simulink model "cambridge"  (R2023b)
settings: Solver=VariableStepAuto  StartTime=0.0  StopTime=15  FixedStep=0.0025  RelTol=1e-3
undefined symbols (not defined in the file or in its folder): body, ctrl, ground, planner, X, Y, Z
libraries: nesl_utility x71, sm_lib x43, slpidlib x24, simulink_extras x12, simulink x8, Contact_Forces_Lib x4, Parts_Lib x4, dspstat3 x1
(part 1 of 6)
settings Model: Creator=biorobotics  LastModifiedBy=Dayan-pc
settings SolverCC: AlgebraicLoopSolver=TrustRegion
settings DataIOCC: ReturnWorkspaceOutputs=off
settings OptimizationCC: ReuseModelBlockBuffer=off
settings DebuggingCC: UnconnectedInputMsg=warning  UnconnectedOutputMsg=warning  UnconnectedLineMsg=warning  ArithmeticOperatorsInVariantConditions=warning
settings ModelReferenceCC: EnableRefExpFcnMdlSchedulingChecks=on
settings SFSimCC: SimUseLocalCustomCode=off  CustomCodeUndefinedFunction=UseInterfaceOnly
settings RTWCC: RTWUseLocalCustomCode=off
settings DiagnosticsConfigSet: SimMechanicsRigidlyBoundBlock=none
settings ExplorerConfigSet: InternalSimMechanicsExplorerSettings="<ExplorerConfiguration><canonicalview>default</canonicalview><AnimationSetting><BasePlaybackSpeed>1.0</BasePlaybackSpeed><PlaybackSpeedFactor>1.0</PlaybackSpeedFactor></AnimationSetting><TilePanel><TileInfo><Tiles Columns=\"1\" Count=\"1\" Rows=\"1\"><Column Weight=\"1\"/><Row Weight=\"1\"/><Tile Height=\"1\" Width=\"1\" X=\"0\" Y=\"0\"/></Tiles></TileInfo><SceneInfo><SceneViewer><BGColor><R>0.60000002384185791</R><G>0.60000002384185791</G><B>0.60000002384185791</B></BGColor><Camera><DoPerspective>off</DoPerspective><Position><X>0</X><Y>-8.51131485710144098</Y><Z>0.265035197138786316</Z></Position><Center><X>0</X><Y>-1.14440917242664142e-07</Y><Z>0.265035197138786316</Z></Center><Up><X>0</X><Y>-0</Y><Z>1</Z></Up><ViewLimDist>1</ViewLimDist><YLim>8.00037523452157551</YLim><XLim>6.17999999999999972</XLim></Camera></SceneViewer></SceneInfo></TilePanel><MechEditorPanel><Cameras/><GfxPanelCameraMap/><VideoCreator><PlaybackSpeedRatio>1.0</PlaybackSpeedRatio><FrameRate>30</FrameRate><VideoFormat>Motion JPEG AVI</VideoFormat><FrameSize>auto</FrameSize></VideoCreator></MechEditorPanel></ExplorerConfiguration>"

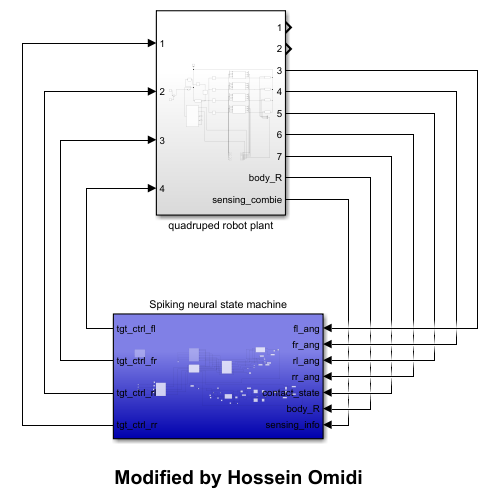
[thumbnail: Simulink's stored preview of the top-level diagram]
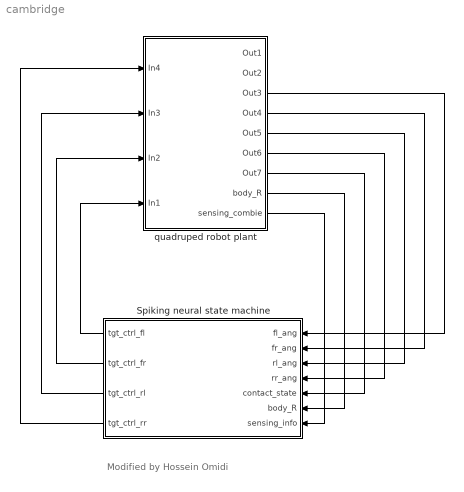
== system cambridge ==
  note: Modified by Hossein Omidi
  Spiking neural state machine : Subsystem
  quadruped robot plant : Subsystem
  wires:
  Spiking neural state machine/1(tgt_ctrl_fl) -> quadruped robot plant/4(In1)
  Spiking neural state machine/2(tgt_ctrl_fr) -> quadruped robot plant/3(In2)
  Spiking neural state machine/3(tgt_ctrl_rl) -> quadruped robot plant/2(In3)
  Spiking neural state machine/4(tgt_ctrl_rr) -> quadruped robot plant/1(In4)
  quadruped robot plant/3(Out3) -> Spiking neural state machine/1(fl_ang)
  quadruped robot plant/4(Out4) -> Spiking neural state machine/2(fr_ang)
  quadruped robot plant/5(Out5) -> Spiking neural state machine/3(rl_ang)
  quadruped robot plant/6(Out6) -> Spiking neural state machine/4(rr_ang)
  quadruped robot plant/7(Out7) -> Spiking neural state machine/5(contact_state)
  quadruped robot plant/8(body_R) -> Spiking neural state machine/6(body_R)
  quadruped robot plant/9(sensing_combie) -> Spiking neural state machine/7(sensing_info)

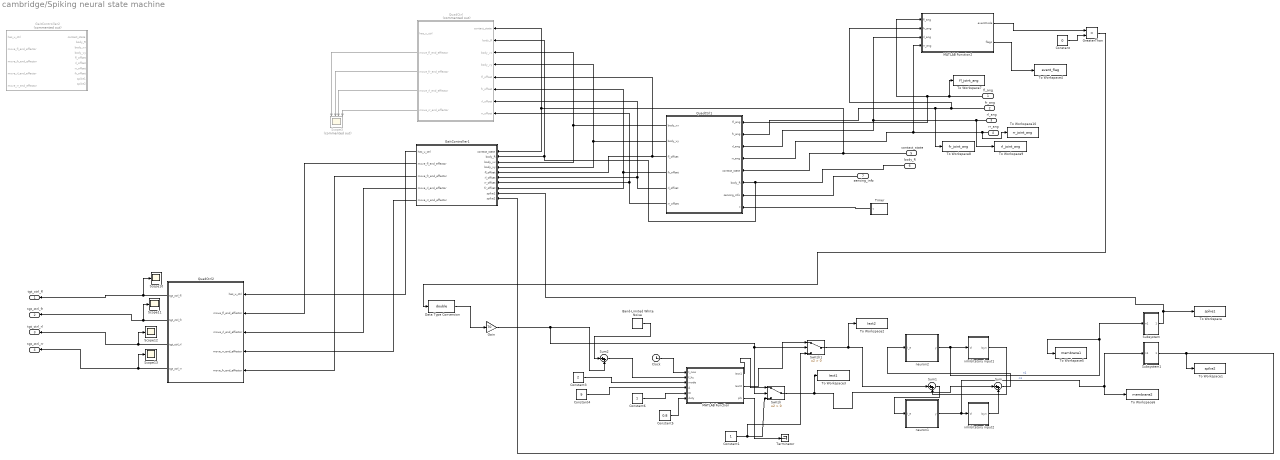
== system cambridge/Spiking neural state machine ==
  fl_ang : Inport
  fr_ang : Inport  Port=2
  rl_ang : Inport  Port=3
  rr_ang : Inport  Port=4
  contact_state : Inport  Port=5
  body_R : Inport  Port=6
  sensing_info : Inport  Port=7
  Band-Limited White Noise : simulink/Sources/Band-Limited White Noise  Cov=[0.1]  Ts=0.1  seed=[23341]
  Clock : Clock
  Constant : Constant  Value=0
  Constant1 : Constant
  Constant3 : Constant  Value=2
  Constant4 : Constant  Value=9
  Constant5 : Constant  Value=0.8
  Constant6 : Constant
  Data Type Conversion : DataTypeConversion  OutDataTypeStr=double  SaturateOnIntegerOverflow=off  RndMeth=Floor
  Gain : Gain  Gain=70
  GaitController1 : Stateflow chart  InitFcn=|  TreatAsAtomicUnit=on
      | % tick timers
      | timer  = uint16(0);
      | timer2 = uint16(0);
      | 
      | % shoulder offsets (body frame)
      | fl_offset = [ body.shoulder_distance;  body.y_length/2 + body.shoulder_size/2; 0 ];
      | fr_offset = [ body.shoulder_distance; -body.y_length/2 - body.shoulder_size/2; 0 ];
      | rl_offset = [-body.shoulder_distance;  body.y_length/2 + body.shoulder_size/2; 0 ];
      | rr_offset = [-body.shoulder_distance; -body.y_length/2 - body.shoulder_size/2; 0 ];
      | 
      | % nominal virtual legs (body frame)
      | vleg1_n = [0;0;planner.stand_height];
      | vleg2_n = [0;0;planner.stand_height];
      | 
      | % swing timing in ticks
      | t_leg    = uint16(planner.leg_swing_time);
      | half_leg = uint16(floor(double(t_leg)/2));
      | 
      | % safe IK inputs on first tick
      | mv_fl = vleg1_n; mv_rr = vleg1_n;
      | mv_fr = vleg2_n; mv_rl = vleg2_n;
      | has_u_ctrl = [1;1;1;1];
  GaitController2 : Stateflow chart  Commented=on  InitFcn=|  TreatAsAtomicUnit=on
      | % tick timers
      | timer  = uint16(0);
      | timer2 = uint16(0);
      | 
      | % shoulder offsets (body frame)
      | fl_offset = [ body.shoulder_distance;  body.y_length/2 + body.shoulder_size/2; 0 ];
      | fr_offset = [ body.shoulder_distance; -body.y_length/2 - body.shoulder_size/2; 0 ];
      | rl_offset = [-body.shoulder_distance;  body.y_length/2 + body.shoulder_size/2; 0 ];
      | rr_offset = [-body.shoulder_distance; -body.y_length/2 - body.shoulder_size/2; 0 ];
      | 
      | % nominal virtual legs (body frame)
      | vleg1_n = [0;0;planner.stand_height];
      | vleg2_n = [0;0;planner.stand_height];
      | 
      | % swing timing in ticks
      | t_leg    = uint16(planner.leg_swing_time);
      | half_leg = uint16(floor(double(t_leg)/2));
      | 
      | % safe IK inputs on first tick
      | mv_fl = vleg1_n; mv_rr = vleg1_n;
      | mv_fr = vleg2_n; mv_rl = vleg2_n;
      | has_u_ctrl = [1;1;1;1];
  GreaterThan : RelationalOperator  Operator=>  OutDataTypeStr=boolean  RndMeth=Simplest  InputSameDT=off
  MATLAB Function : MATLAB Function  TreatAsAtomicUnit=on
  MATLAB Function2 : MATLAB Function  TreatAsAtomicUnit=on
  QuadCtrl : MATLAB Function  Commented=on  TreatAsAtomicUnit=on  SystemSampleTime=0.0025
  QuadCtrl1 : MATLAB Function  TreatAsAtomicUnit=on  SystemSampleTime=0.0025
  QuadCtrl2 : MATLAB Function  TreatAsAtomicUnit=on  SystemSampleTime=0.0025
  Scope{10..13} (4 alike) : Scope
  Scope3 : Scope  Commented=on  NumInputPorts=4
  Subsystem : Subsystem
  Subsystem1 : Subsystem
  Sum : Sum  Inputs=|++
  Sum1 : Sum  Inputs=|++
  Sum2 : Sum  Inputs=|++
  Switch : Switch  Criteria=u2 > Threshold  SaturateOnIntegerOverflow=off  InputSameDT=off
  Switch1 : Switch  Criteria=u2 > Threshold  SaturateOnIntegerOverflow=off  InputSameDT=off
  Terminator : Terminator
  Timer : Subsystem
  To Workspace : ToWorkspace  VariableName=spike1  SaveFormat=Timeseries  SampleTime=-1
  To Workspace1 : ToWorkspace  VariableName=spike2  SaveFormat=Timeseries  SampleTime=-1
  To Workspace10 : ToWorkspace  VariableName=rr_joint_ang  SaveFormat=Timeseries  SampleTime=-1
  To Workspace2 : ToWorkspace  VariableName=Iext2  SaveFormat=Timeseries  SampleTime=-1
  To Workspace3 : ToWorkspace  VariableName=Iext1  SaveFormat=Timeseries  SampleTime=-1
  To Workspace4 : ToWorkspace  VariableName=event_flag  SaveFormat=Timeseries  SampleTime=-1
  To Workspace5 : ToWorkspace  VariableName=membrane1  SaveFormat=Timeseries  SampleTime=-1
  To Workspace6 : ToWorkspace  VariableName=membrane2  SaveFormat=Timeseries  SampleTime=-1
  To Workspace7 : ToWorkspace  VariableName=fl_joint_ang  SaveFormat=Timeseries  SampleTime=-1
  To Workspace8 : ToWorkspace  VariableName=fr_joint_ang  SaveFormat=Timeseries  SampleTime=-1
  To Workspace9 : ToWorkspace  VariableName=rl_joint_ang  SaveFormat=Timeseries  SampleTime=-1
  inhibitatory input1 : Subsystem
  inhibitatory input2 : Subsystem
  neuron1 : Subsystem
  neuron2 : Subsystem
  tgt_ctrl_fl : Outport  VectorParamsAs1DForOutWhenUnconnected=off
  tgt_ctrl_fr : Outport  Port=2  VectorParamsAs1DForOutWhenUnconnected=off
  tgt_ctrl_rl : Outport  Port=3  VectorParamsAs1DForOutWhenUnconnected=off
  tgt_ctrl_rr : Outport  Port=4  VectorParamsAs1DForOutWhenUnconnected=off
  wires:
  Timer/1(t) -> QuadCtrl1/8(t)
  fl_ang/1 -> To Workspace7/1, MATLAB Function2/1(fl_ang), QuadCtrl1/1(fl_ang)
  fr_ang/1 -> To Workspace8/1, QuadCtrl1/2(fr_ang), MATLAB Function2/2(fr_ang)
  rl_ang/1 -> To Workspace9/1, MATLAB Function2/3(rl_ang), QuadCtrl1/3(rl_ang)
  rr_ang/1 -> To Workspace10/1, MATLAB Function2/4(rr_ang), QuadCtrl1/4(rr_ang)
  sensing_info/1 -> QuadCtrl1/7(sensing_info)
  QuadCtrl2/1(tgt_ctrl_fl) -> Scope10/1, tgt_ctrl_fl/1
  QuadCtrl2/2(tgt_ctrl_fr) -> Scope11/1, tgt_ctrl_fr/1
  QuadCtrl2/3(tgt_ctrl_rl) -> Scope12/1, tgt_ctrl_rl/1
  QuadCtrl2/4(tgt_ctrl_rr) -> Scope13/1, tgt_ctrl_rr/1
  contact_state/1 -> QuadCtrl/1(contact_state), GaitController1/1(contact_state), QuadCtrl1/5(contact_state)
  body_R/1 -> QuadCtrl/2(body_R), GaitController1/2(body_R), QuadCtrl1/6(body_R)
  QuadCtrl1/1(body_vx) -> QuadCtrl/3(body_vx), GaitController1/3(body_vx)
  QuadCtrl1/2(body_vy) -> QuadCtrl/4(body_vy), GaitController1/4(body_vy)
  QuadCtrl1/3(fl_offset) -> QuadCtrl/5(fl_offset), GaitController1/5(fl_offset)
  QuadCtrl1/5(rl_offset) -> QuadCtrl/7(rl_offset), GaitController1/6(rl_offset)
  QuadCtrl1/6(rr_offset) -> QuadCtrl/8(rr_offset), GaitController1/7(rr_offset)
  QuadCtrl1/4(fr_offset) -> QuadCtrl/6(fr_offset), GaitController1/8(fr_offset)
  GaitController1/1(has_u_ctrl) -> QuadCtrl2/1(has_u_ctrl)
  GaitController1/2(move_fl_end_effector) -> QuadCtrl2/2(move_fl_end_effector)
  GaitController1/3(move_fr_end_effector) -> QuadCtrl2/5(move_fr_end_effector)
  GaitController1/4(move_rl_end_effector) -> QuadCtrl2/3(move_rl_end_effector)
  GaitController1/5(move_rr_end_effector) -> QuadCtrl2/4(move_rr_end_effector)
  QuadCtrl/2(move_fl_end_effector) -> Scope3/1
  QuadCtrl/3(move_fr_end_effector) -> Scope3/2
  QuadCtrl/4(move_rl_end_effector) -> Scope3/3
  QuadCtrl/5(move_rr_end_effector) -> Scope3/4
  MATLAB Function2/2(flags) -> To Workspace4/1
  Constant3/1 -> MATLAB Function/3(mode)
  Gain/1 -> Sum2/2, Switch1/2, Switch/2
  Clock/1 -> MATLAB Function/1(t_now)
  inhibitatory input2/1(Isyn) -> Sum/2
  Constant5/1 -> MATLAB Function/6(duty)
  inhibitatory input1/1(Isyn) -> Sum1/2
  Constant4/1 -> MATLAB Function/4(A)
  Constant6/1 -> MATLAB Function/5(I0)
  Subsystem1/1(spike2) -> To Workspace1/1, GaitController1/10(spike2)
  Sum/1 -> neuron2/1(I_e)
  neuron2/1(y) -> Subsystem/1(n1), To Workspace5/1, inhibitatory input1/1(Vi)  "n1"
  MATLAB Function/2(Iext2) -> Switch1/1
  neuron1/1(y) -> Subsystem1/1(n1), To Workspace6/1, inhibitatory input2/1(Vi)  "n1"
  Sum1/1 -> neuron1/1(I_e)
  MATLAB Function/1(Iext1) -> Switch/1
  MATLAB Function2/1(eventCode) -> GreaterThan/1
  Constant/1 -> GreaterThan/2
  Data Type Conversion/1 -> Gain/1
  GreaterThan/1 -> Data Type Conversion/1
  Switch/1 -> To Workspace3/1, Sum/1
  Constant1/1 -> Switch1/3, Switch/3
  Switch1/1 -> To Workspace2/1, Sum1/1
  Subsystem/1(Out1) -> To Workspace/1, GaitController1/9(spike1)
  Band-Limited White Noise/1 -> Sum2/1
  Sum2/1 -> MATLAB Function/2(f_hz)
  MATLAB Function/3(phi) -> Terminator/1

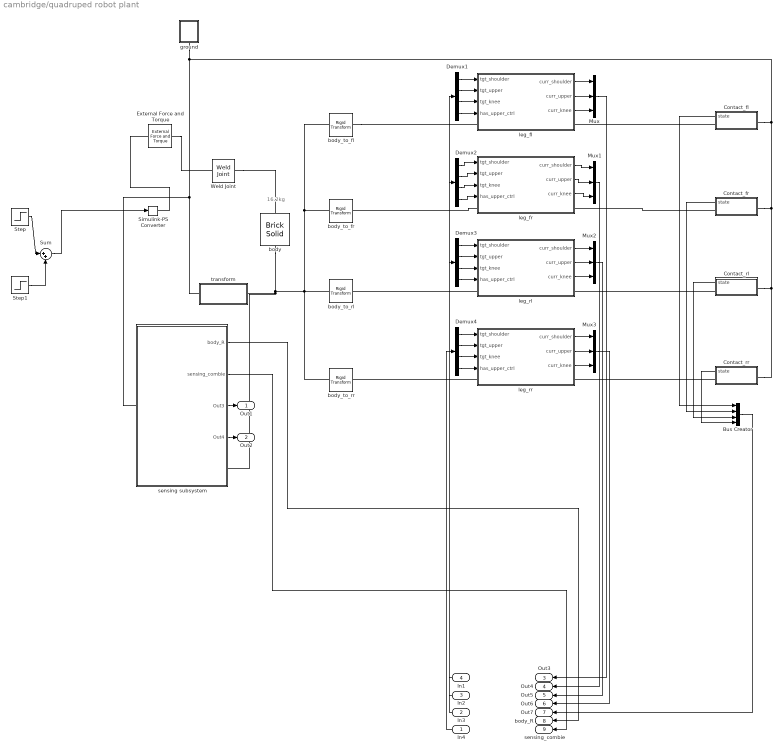
== system cambridge/quadruped robot plant ==
  note: 16.2kg
  In4 : Inport
  In3 : Inport  Port=2
  In2 : Inport  Port=3
  In1 : Inport  Port=4
  Bus Creator : BusCreator  Inputs=4
  Contact_fl : Subsystem
  Contact_fr : Subsystem
  Contact_rl : Subsystem
  Contact_rr : Subsystem
  Demux{1..4} (4 alike) : Demux
  External Force and Torque : sm_lib/Forces and Torques/External Force and Torque  ForceResolutionFrame=AttachedFrame  EnableForceX=on  EnableForceY=off  EnableForceZ=off  EnableForce=off  TorqueResolutionFrame=AttachedFrame  EnableTorqueX=off  EnableTorqueY=off  EnableTorqueZ=off  EnableTorque=off
  Mux{,1..3} (4 alike) : Mux  Inputs=3
  Simulink-PS Converter : nesl_utility/Simulink-PS Converter  PhysicalDomain=network_engine_domain  SubClassName=ps_input  LeftPortType=input  RightPortType=output  PseudoPeriodic=off  Frequencies=[]  NoiseDistribution=none  NoiseParameters=[]  Unit=1  AffineConversion=off  FilteringAndDerivatives=provide  SimscapeFilterOrder=1  InputFilterTimeConstant=0.001  UdotUserProvided=0
  Step : Step  Time=5  After=100  SampleTime=0
  Step1 : Step  Time=5.1  After=-100  SampleTime=0
  Sum : Sum  Inputs=|++
  Weld Joint : sm_lib/Joints/Weld Joint  JointMode=Normal  SenseConstraintForce=off  SenseConstraintForceX=off  SenseConstraintForceY=off  SenseConstraintForceZ=off  SenseConstraintTorque=off  SenseConstraintTorqueX=off  SenseConstraintTorqueY=off  SenseConstraintTorqueZ=off  SenseTotalForce=off  SenseTotalForceX=off  SenseTotalForceY=off  SenseTotalForceZ=off  SenseTotalTorque=off  SenseTotalTorqueX=off  SenseTotalTorqueY=off  SenseTotalTorqueZ=off  CompositeWrenchDir=FollowerOnBase  CompositeWrenchFrame=BaseFrame
  body : sm_lib/Body Elements/Brick Solid  GraphicAmbientColor=[0.15 0.15 0.15 1.0]  BasedOnType=Density  BrickDimensions=[body.x_length body.y_length body.z_length]  BrickDimensionsUnits=m  CenterOfMass=[0 0 0]  CenterOfMassUnits=m  GraphicDiffuseColor=[1.0 0.0 0.2]  Density=600  DensityUnits=kg/(m^3)  DoExposeReferenceFrame=on  GraphicEmissiveColor=[0.0 0.0 0.0 1.0]  ExportEntireGeometry=off  SerializedFrames=<Frames><Frame><Id>Frame2</Id><Value><Name>force</Name><Origin><Source>CenterOfMassFrame</Source><FeatureName></FeatureName></Origin><PrimaryAxis><DefinedDirection>+Z</DefinedDirection><Source>ReferenceFrame</Source><SourceDirection>+Z</SourceDirection><FeatureName></FeatureName></PrimaryAxis><SecondaryAxis><DefinedDirection>+X</DefinedDirection><Source>ReferenceFrame</Source><SourceDirection>+X</SourceDirection><FeatureName></FeatureName></SecondaryAxis></Value></Frame></Frames>  MarkerShape=Sphere  MarkerSize=10  GraphicType=FromGeometry  InertiaType=CalculateFromGeometry  Mass=8.6  MassUnits=kg  MomentsOfInertia=[1 1 1]  MomentsOfInertiaUnits=kg*m^2  GraphicOpacity=1.0  ProductsOfInertia=[0 0 0]  ProductsOfInertiaUnits=kg*m^2  GraphicShininess=75  GraphicSpecularColor=[0.5 0.5 0.5 1.0]  GraphicVisPropType=SimpleVisualProperties
  body_to_fl : sm_lib/Frames and Transforms/Rigid Transform  TranslationMethod=Cartesian  TranslationStandardOffset=0  TranslationStandardOffsetUnits=m  TranslationStandardAxis=+Z  TranslationCartesianOffset=[body.shoulder_distance body.y_length/2+body.shoulder_size/2 0]  TranslationCartesianOffsetUnits=m  TranslationROffset=0  TranslationROffsetUnits=m  TranslationZOffset=0  TranslationZOffsetUnits=m  TranslationThetaOffset=0  TranslationThetaOffsetUnits=deg  RotationMethod=AlignedAxes  RotationAngleUnits=deg  RotationStandardAxis=+Z  RotationAngle=0.0  RotationArbitraryAxis=[0 0 1]  FollAlignAxisA=+Z  BaseAlignAxisA=+X  FollAlignAxisB=+X  BaseAlignAxisB=-Z  RotationSequenceAxes=FollowerAxes  RotationSequence=XYX  RotationSequenceAngles=[0 0 0]  RotationSequenceAnglesUnits=deg  RotationMatrix=[1 0 0; 0 1 0; 0 0 1]  Quaternion=[1 0 0 0]
  body_to_fr : sm_lib/Frames and Transforms/Rigid Transform  TranslationMethod=Cartesian  TranslationStandardOffset=0  TranslationStandardOffsetUnits=m  TranslationStandardAxis=+Z  TranslationCartesianOffset=[body.shoulder_distance -body.y_length/2-body.shoulder_size/2 0]  TranslationCartesianOffsetUnits=m  TranslationROffset=0  TranslationROffsetUnits=m  TranslationZOffset=0  TranslationZOffsetUnits=m  TranslationThetaOffset=0  TranslationThetaOffsetUnits=deg  RotationMethod=AlignedAxes  RotationAngleUnits=deg  RotationStandardAxis=+Z  RotationAngle=0.0  RotationArbitraryAxis=[0 0 1]  FollAlignAxisA=+Z  BaseAlignAxisA=+X  FollAlignAxisB=+X  BaseAlignAxisB=-Z  RotationSequenceAxes=FollowerAxes  RotationSequence=XYX  RotationSequenceAngles=[0 0 0]  RotationSequenceAnglesUnits=deg  RotationMatrix=[1 0 0; 0 1 0; 0 0 1]  Quaternion=[1 0 0 0]
  body_to_rl : sm_lib/Frames and Transforms/Rigid Transform  TranslationMethod=Cartesian  TranslationStandardOffset=0  TranslationStandardOffsetUnits=m  TranslationStandardAxis=+Z  TranslationCartesianOffset=[-body.shoulder_distance body.y_length/2+body.shoulder_size/2 0]  TranslationCartesianOffsetUnits=m  TranslationROffset=0  TranslationROffsetUnits=m  TranslationZOffset=0  TranslationZOffsetUnits=m  TranslationThetaOffset=0  TranslationThetaOffsetUnits=deg  RotationMethod=AlignedAxes  RotationAngleUnits=deg  RotationStandardAxis=+Z  RotationAngle=0.0  RotationArbitraryAxis=[0 0 1]  FollAlignAxisA=+Z  BaseAlignAxisA=+X  FollAlignAxisB=+X  BaseAlignAxisB=-Z  RotationSequenceAxes=FollowerAxes  RotationSequence=XYX  RotationSequenceAngles=[0 0 0]  RotationSequenceAnglesUnits=deg  RotationMatrix=[1 0 0; 0 1 0; 0 0 1]  Quaternion=[1 0 0 0]
  body_to_rr : sm_lib/Frames and Transforms/Rigid Transform  TranslationMethod=Cartesian  TranslationStandardOffset=0  TranslationStandardOffsetUnits=m  TranslationStandardAxis=+Z  TranslationCartesianOffset=[-body.shoulder_distance -body.y_length/2-body.shoulder_size/2 0]  TranslationCartesianOffsetUnits=m  TranslationROffset=0  TranslationROffsetUnits=m  TranslationZOffset=0  TranslationZOffsetUnits=m  TranslationThetaOffset=0  TranslationThetaOffsetUnits=deg  RotationMethod=AlignedAxes  RotationAngleUnits=deg  RotationStandardAxis=+Z  RotationAngle=0.0  RotationArbitraryAxis=[0 0 1]  FollAlignAxisA=+Z  BaseAlignAxisA=+X  FollAlignAxisB=+X  BaseAlignAxisB=-Z  RotationSequenceAxes=FollowerAxes  RotationSequence=XYX  RotationSequenceAngles=[0 0 0]  RotationSequenceAnglesUnits=deg  RotationMatrix=[1 0 0; 0 1 0; 0 0 1]  Quaternion=[1 0 0 0]
  ground : Subsystem
  leg_fl : Subsystem
  leg_fr : Subsystem
  leg_rl : Subsystem
  leg_rr : Subsystem
  "sensing subsystem " : Subsystem
  transform : Subsystem
  Out1 : Outport
  Out2 : Outport  Port=2
  Out3 : Outport  Port=3
  Out4 : Outport  Port=4
  Out5 : Outport  Port=5
  Out6 : Outport  Port=6
  Out7 : Outport  Port=7
  body_R : Outport  Port=8
  sensing_combie : Outport  Port=9
  wires:
  Bus Creator/1 -> Out7/1
  Demux2/1 -> leg_fr/1(tgt_shoulder)
  Demux1/2 -> leg_fl/2(tgt_upper)
  Demux2/3 -> leg_fr/3(tgt_knee)
  Demux4/4 -> leg_rr/4(has_upper_ctrl)
  "sensing subsystem "/1(body_R) -> body_R/1
  leg_rr/1(curr_shoulder) -> Mux3/1
  Sum/1 -> Simulink-PS Converter/1
  Demux3/4 -> leg_rl/4(has_upper_ctrl)
  Demux2/2 -> leg_fr/2(tgt_upper)
  Demux3/1 -> leg_rl/1(tgt_shoulder)
  Demux3/3 -> leg_rl/3(tgt_knee)
  Mux/1 -> Out3/1
  Contact_rl/1(state) -> Bus Creator/3
  leg_rl/2("curr_upper ") -> Mux2/2
  Demux4/3 -> leg_rr/3(tgt_knee)
  leg_fl/3(curr_knee) -> Mux/3
  leg_fl/1(curr_shoulder) -> Mux/1
  Step1/1 -> Sum/2
  leg_fr/3(curr_knee) -> Mux1/3
  leg_fr/1(curr_shoulder) -> Mux1/1
  leg_rl/1(curr_shoulder) -> Mux2/1
  Contact_fr/1(state) -> Bus Creator/2
  Demux4/1 -> leg_rr/1(tgt_shoulder)
  Demux1/4 -> leg_fl/4(has_upper_ctrl)
  leg_fl/2("curr_upper ") -> Mux/2
  Demux2/4 -> leg_fr/4(has_upper_ctrl)
  "sensing subsystem "/4(Out4) -> Out2/1
  Mux1/1 -> Out4/1
  Contact_fl/1(state) -> Bus Creator/1
  leg_rr/2("curr_upper ") -> Mux3/2
  leg_rr/3(curr_knee) -> Mux3/3
  In1/1 -> Demux1/1
  Demux1/1 -> leg_fl/1(tgt_shoulder)
  Step/1 -> Sum/1
  leg_rl/3(curr_knee) -> Mux2/3
  Demux3/2 -> leg_rl/2(tgt_upper)
  Demux1/3 -> leg_fl/3(tgt_knee)
  Demux4/2 -> leg_rr/2(tgt_upper)
  In3/1 -> Demux3/1
  Contact_rr/1(state) -> Bus Creator/4
  leg_fr/2("curr_upper ") -> Mux1/2
  Mux3/1 -> Out6/1
  Mux2/1 -> Out5/1
  "sensing subsystem "/2(sensing_combie) -> sensing_combie/1
  In2/1 -> Demux2/1
  In4/1 -> Demux4/1
  "sensing subsystem "/3(Out3) -> Out1/1
  connections:
  body_to_fl/LConn1 -- "sensing subsystem "/RConn1 -- transform/LConn1 -- body/RConn1 -- body_to_rr/LConn1 -- body_to_rl/LConn1 -- body_to_fr/LConn1
  Contact_rl/RConn1 -- leg_rl/RConn1
  External Force and Torque/RConn1 -- Weld Joint/LConn1
  leg_fr/LConn1 -- body_to_fr/RConn1
  Contact_fr/RConn1 -- leg_fr/RConn1
  External Force and Torque/LConn1 -- Simulink-PS Converter/RConn1
  Contact_fr/LConn1 -- "sensing subsystem "/LConn1 -- transform/RConn1 -- ground/RConn1 -- Contact_fl/LConn1 -- Contact_rr/LConn1 -- Contact_rl/LConn1
  leg_rr/LConn1 -- body_to_rr/RConn1
  body_to_fl/RConn1 -- leg_fl/LConn1
  Contact_rr/RConn1 -- leg_rr/RConn1
  leg_rl/LConn1 -- body_to_rl/RConn1
  Contact_fl/RConn1 -- leg_fl/RConn1
  Weld Joint/RConn1 -- body/LConn1

== system cambridge/Spiking neural state machine/Subsystem ==
  n1 : Inport
  AND : Logic  IconShape=distinctive  AllPortsSameDT=off  OutDataTypeStr=boolean
  Constant2 : Constant
  Detect Rise Positive : simulink/Logic and Bit Operations/Detect Rise Positive  vinit=0  OutDataTypeStr=boolean
  GreaterThan1 : RelationalOperator  Operator=>  OutDataTypeStr=boolean  RndMeth=Simplest  InputSameDT=off
  Out1 : Outport
  wires:
  AND/1 -> Out1/1
  n1/1 -> Detect Rise Positive/1, GreaterThan1/1
  Constant2/1 -> GreaterThan1/2
  Detect Rise Positive/1 -> AND/1
  GreaterThan1/1 -> AND/2

== system cambridge/Spiking neural state machine/Subsystem1 ==
  n1 : Inport
  AND : Logic  IconShape=distinctive  AllPortsSameDT=off  OutDataTypeStr=boolean
  Constant2 : Constant
  Detect Rise Positive : simulink/Logic and Bit Operations/Detect Rise Positive  vinit=0  OutDataTypeStr=boolean
  GreaterThan1 : RelationalOperator  Operator=>  OutDataTypeStr=boolean  RndMeth=Simplest  InputSameDT=off
  spike2 : Outport
  wires:
  GreaterThan1/1 -> AND/2
  Detect Rise Positive/1 -> AND/1
  Constant2/1 -> GreaterThan1/2
  n1/1 -> GreaterThan1/1, Detect Rise Positive/1
  AND/1 -> spike2/1

== system cambridge/Spiking neural state machine/Timer ==
  Compare To Constant : simulink/Logic and Bit Operations/Compare To Constant  relop=>=  const=planner.time_circle  OutDataTypeStr=boolean
  Constant4 : Constant
  Integrator : Integrator  ExternalReset=level
  Memory : Memory
  t : Outport  VectorParamsAs1DForOutWhenUnconnected=off
  wires:
  Constant4/1 -> Integrator/1
  Integrator/1 -> Memory/1, t/1
  Compare To Constant/1 -> Integrator/2
  Memory/1 -> Compare To Constant/1

== system cambridge/Spiking neural state machine/inhibitatory input1 ==
  Vi : Inport
  Constant1 : Constant
  Constant2 : Constant  Value=-65
  Constant3 : Constant  Value=-10
  Constant4 : Constant  Value=1.5
  Integrator : Integrator
  MATLAB Function : MATLAB Function  TreatAsAtomicUnit=on
  MATLAB Function1 : MATLAB Function  TreatAsAtomicUnit=on
  Isyn : Outport
  wires:
  MATLAB Function1/1(Isyn) -> Isyn/1
  Constant1/1 -> MATLAB Function/3(tau)
  Constant4/1 -> MATLAB Function1/4(alpha)
  MATLAB Function/1(dVf) -> Integrator/1
  Integrator/1 -> MATLAB Function1/1(Vf), MATLAB Function/1(Vf)
  Vi/1 -> MATLAB Function/2(Vi)
  Constant3/1 -> MATLAB Function1/3(gsyn)
  Constant2/1 -> MATLAB Function1/2(Vth)

== system cambridge/Spiking neural state machine/inhibitatory input2 ==
  Vi : Inport
  Constant1 : Constant
  Constant2 : Constant  Value=-65
  Constant3 : Constant  Value=-10
  Constant4 : Constant  Value=1.5
  Integrator : Integrator
  MATLAB Function : MATLAB Function  TreatAsAtomicUnit=on
  MATLAB Function1 : MATLAB Function  TreatAsAtomicUnit=on
  Isyn : Outport
  wires:
  Constant2/1 -> MATLAB Function1/2(Vth)
  Constant3/1 -> MATLAB Function1/3(gsyn)
  Vi/1 -> MATLAB Function/2(Vi)
  Integrator/1 -> MATLAB Function/1(Vf), MATLAB Function1/1(Vf)
  MATLAB Function/1(dVf) -> Integrator/1
  Constant4/1 -> MATLAB Function1/4(alpha)
  Constant1/1 -> MATLAB Function/3(tau)
  MATLAB Function1/1(Isyn) -> Isyn/1

== system cambridge/Spiking neural state machine/neuron1 ==
  I_e : Inport
  Demux : Demux
  Demux1 : Demux
  Integrator : Integrator  InitialCondition=[-65; 0.05; 0.60; 0.32]
  MATLAB Function : MATLAB Function  TreatAsAtomicUnit=on
  Mux : Mux
  Terminator : Terminator
  Terminator1 : Terminator
  Terminator2 : Terminator
  y : Outport
  wires:
  Demux1/1 -> y/1
  Demux1/2 -> Terminator2/1
  Demux1/3 -> Terminator1/1
  Demux1/4 -> Terminator/1
  I_e/1 -> MATLAB Function/5(I_e)
  MATLAB Function/2(dm) -> Mux/2
  Demux/4 -> MATLAB Function/4(n)
  Demux/2 -> MATLAB Function/2(m)
  Demux/3 -> MATLAB Function/3(h)
  Integrator/1 -> Demux1/1, Demux/1  "y"
  MATLAB Function/4(dn) -> Mux/4
  MATLAB Function/3(dh) -> Mux/3
  Demux/1 -> MATLAB Function/1(v)
  Mux/1 -> Integrator/1  "dy"
  MATLAB Function/1(dv) -> Mux/1

== system cambridge/Spiking neural state machine/neuron2 ==
  I_e : Inport
  Demux : Demux
  Demux1 : Demux
  Integrator : Integrator  InitialCondition=[-65; 0.05; 0.60; 0.32]
  MATLAB Function : MATLAB Function  TreatAsAtomicUnit=on
  Mux : Mux
  Terminator : Terminator
  Terminator1 : Terminator
  Terminator2 : Terminator
  y : Outport
  wires:
  MATLAB Function/1(dv) -> Mux/1
  Mux/1 -> Integrator/1  "dy"
  Demux/1 -> MATLAB Function/1(v)
  MATLAB Function/3(dh) -> Mux/3
  MATLAB Function/4(dn) -> Mux/4
  Integrator/1 -> Demux/1, Demux1/1  "y"
  Demux/3 -> MATLAB Function/3(h)
  Demux/2 -> MATLAB Function/2(m)
  Demux/4 -> MATLAB Function/4(n)
  MATLAB Function/2(dm) -> Mux/2
  I_e/1 -> MATLAB Function/5(I_e)
  Demux1/4 -> Terminator/1
  Demux1/3 -> Terminator1/1
  Demux1/2 -> Terminator2/1
  Demux1/1 -> y/1

== system cambridge/quadruped robot plant/Contact_fl ==
  note: state 4 166.31ms
  note: 这是一个蛋疼的处理，因为地面现在厚度是0.4，为了和碰撞的block要求匹配，所以碰撞是相对于这个地面的中心来算的。而检测高度的时候就要把这个厚度减掉
      | 但是Transform sensor要检测的是球和地面的高度差
  Bus Selector : BusSelector  OutputSignals=Normal Force,Frame Sep,Friction Force
  Compare To Constant : simulink/Logic and Bit Operations/Compare To Constant  relop=<=  const=planner.touch_down_height  OutDataTypeStr=uint8
  PSConv4 : nesl_utility/PS-Simulink Converter  PhysicalDomain=network_engine_domain  SubClassName=ps_output  LeftPortType=input  RightPortType=output  PseudoPeriodic=off  Frequencies=[]  VectorFormat=1-D array  Unit=1  AffineConversion=off
  Sphere to Plane Force1 : Contact_Forces_Lib/3D/Sphere to Plane Force  sphere_rad=body.foot_radius  plane_lenx=12  plane_leny=12  plane_depth=0  force_law=Linear  k_contact=ground.stiff  b_contact=ground.damp  pen_full_damp_F=1e-4  pen_exponent=1  custom_param_1=1  custom_param_2=1  friction_law=Stick-Slip Continuous  mu_kinetic=0.7  mu_static=0.7  v_thr=0.001
  State Scope : Scope
  Terminator : Terminator
  Transform Sensor : sm_lib/Frames and Transforms/Transform Sensor  MeasurementFrame=World  RotationSequence=XYX  SenseAngle=off  SenseAxis=off  SenseQ=off  SenseR=off  SenseRotationSequence=off  SenseOmegaX=off  SenseOmegaY=off  SenseOmegaZ=off  SenseOmega=off  SenseQDot=off  SenseRDot=off  SenseRotationSequenceDot=off  SenseAlphaX=off  SenseAlphaY=off  SenseAlphaZ=off  SenseAlpha=off  SenseQDDot=off  SenseRDDot=off  SenseX=off  SenseY=off  SenseZ=on  SenseXYZ=off  SenseRad=off  SenseAzim=off  SenseDist=off  SenseInc=off  SenseXDot=off  SenseYDot=off  SenseZDot=off  SenseXYZDot=off  SenseRadDot=off  SenseAzimDot=off  SenseDistDot=off  SenseIncDot=off  SenseXDDot=off  SenseYDDot=off  SenseZDDot=off  SenseXYZDDot=off  SenseRadDDot=off  SenseAzimDDot=off  SenseDistDDot=off  SenseIncDDot=off
  ZScope : Scope
  force : Scope  NumInputPorts=2
  PlanB : PMIOPort  Side=Left
  SphF : PMIOPort  Port=2  Side=Right
  state : Outport  VectorParamsAs1DForOutWhenUnconnected=off
  wires:
  Sphere to Plane Force1/1 -> Bus Selector/1
  Bus Selector/1 -> force/1  "<Normal Force>"
  PSConv4/1 -> Compare To Constant/1, ZScope/1
  Compare To Constant/1 -> state/1, State Scope/1
  Bus Selector/3 -> force/2  "<Friction Force>"
  Bus Selector/2 -> Terminator/1  "<Frame Sep>"
  connections:
  Sphere to Plane Force1/LConn1 -- Transform Sensor/RConn1 -- SphF/RConn1
  Sphere to Plane Force1/RConn1 -- Transform Sensor/LConn1 -- PlanB/RConn1
  PSConv4/LConn1 -- Transform Sensor/RConn2

== system cambridge/quadruped robot plant/Contact_fr ==
  note: state 4 166.31ms
  note: 这是一个蛋疼的处理，因为地面现在厚度是0.4，为了和碰撞的block要求匹配，所以碰撞是相对于这个地面的中心来算的。而检测高度的时候就要把这个厚度减掉
      | 但是Transform sensor要检测的是球和地面的高度差
  Bus Selector : BusSelector  OutputSignals=Normal Force,Frame Sep,Friction Force
  Compare To Constant : simulink/Logic and Bit Operations/Compare To Constant  relop=<=  const=planner.touch_down_height  OutDataTypeStr=uint8
  PSConv4 : nesl_utility/PS-Simulink Converter  PhysicalDomain=network_engine_domain  SubClassName=ps_output  LeftPortType=input  RightPortType=output  PseudoPeriodic=off  Frequencies=[]  VectorFormat=1-D array  Unit=1  AffineConversion=off
  Sphere to Plane Force1 : Contact_Forces_Lib/3D/Sphere to Plane Force  sphere_rad=body.foot_radius  plane_lenx=12  plane_leny=12  plane_depth=0  force_law=Linear  k_contact=ground.stiff  b_contact=ground.damp  pen_full_damp_F=1e-4  pen_exponent=1  custom_param_1=1  custom_param_2=1  friction_law=Stick-Slip Continuous  mu_kinetic=0.7  mu_static=0.7  v_thr=0.001
  State Scope : Scope
  Terminator : Terminator
  Transform Sensor : sm_lib/Frames and Transforms/Transform Sensor  MeasurementFrame=World  RotationSequence=XYX  SenseAngle=off  SenseAxis=off  SenseQ=off  SenseR=off  SenseRotationSequence=off  SenseOmegaX=off  SenseOmegaY=off  SenseOmegaZ=off  SenseOmega=off  SenseQDot=off  SenseRDot=off  SenseRotationSequenceDot=off  SenseAlphaX=off  SenseAlphaY=off  SenseAlphaZ=off  SenseAlpha=off  SenseQDDot=off  SenseRDDot=off  SenseX=off  SenseY=off  SenseZ=on  SenseXYZ=off  SenseRad=off  SenseAzim=off  SenseDist=off  SenseInc=off  SenseXDot=off  SenseYDot=off  SenseZDot=off  SenseXYZDot=off  SenseRadDot=off  SenseAzimDot=off  SenseDistDot=off  SenseIncDot=off  SenseXDDot=off  SenseYDDot=off  SenseZDDot=off  SenseXYZDDot=off  SenseRadDDot=off  SenseAzimDDot=off  SenseDistDDot=off  SenseIncDDot=off
  ZScope : Scope
  force : Scope  NumInputPorts=2
  PlanB : PMIOPort  Side=Left
  SphF : PMIOPort  Port=2  Side=Right
  state : Outport  VectorParamsAs1DForOutWhenUnconnected=off
  wires:
  Sphere to Plane Force1/1 -> Bus Selector/1
  Bus Selector/1 -> force/1  "<Normal Force>"
  PSConv4/1 -> Compare To Constant/1, ZScope/1
  Compare To Constant/1 -> state/1, State Scope/1
  Bus Selector/3 -> force/2  "<Friction Force>"
  Bus Selector/2 -> Terminator/1  "<Frame Sep>"
  connections:
  Sphere to Plane Force1/LConn1 -- Transform Sensor/RConn1 -- SphF/RConn1
  Sphere to Plane Force1/RConn1 -- Transform Sensor/LConn1 -- PlanB/RConn1
  PSConv4/LConn1 -- Transform Sensor/RConn2

== system cambridge/quadruped robot plant/Contact_rl ==
  note: 这是一个蛋疼的处理，因为地面现在厚度是0.4，为了和碰撞的block要求匹配，所以碰撞是相对于这个地面的中心来算的。而检测高度的时候就要把这个厚度减掉
      | 但是Transform sensor要检测的是球和地面的高度差
  Bus Selector : BusSelector  OutputSignals=Normal Force,Frame Sep,Friction Force
  Compare To Constant : simulink/Logic and Bit Operations/Compare To Constant  relop=<=  const=planner.touch_down_height  OutDataTypeStr=uint8
  PSConv4 : nesl_utility/PS-Simulink Converter  PhysicalDomain=network_engine_domain  SubClassName=ps_output  LeftPortType=input  RightPortType=output  PseudoPeriodic=off  Frequencies=[]  VectorFormat=1-D array  Unit=1  AffineConversion=off
  Sphere to Plane Force1 : Contact_Forces_Lib/3D/Sphere to Plane Force  sphere_rad=body.foot_radius  plane_lenx=12  plane_leny=12  plane_depth=0  force_law=Linear  k_contact=ground.stiff  b_contact=ground.damp  pen_full_damp_F=1e-4  pen_exponent=1  custom_param_1=1  custom_param_2=1  friction_law=Stick-Slip Continuous  mu_kinetic=0.7  mu_static=0.7  v_thr=0.001
  State Scope : Scope
  Terminator : Terminator
  Transform Sensor : sm_lib/Frames and Transforms/Transform Sensor  MeasurementFrame=World  RotationSequence=XYX  SenseAngle=off  SenseAxis=off  SenseQ=off  SenseR=off  SenseRotationSequence=off  SenseOmegaX=off  SenseOmegaY=off  SenseOmegaZ=off  SenseOmega=off  SenseQDot=off  SenseRDot=off  SenseRotationSequenceDot=off  SenseAlphaX=off  SenseAlphaY=off  SenseAlphaZ=off  SenseAlpha=off  SenseQDDot=off  SenseRDDot=off  SenseX=off  SenseY=off  SenseZ=on  SenseXYZ=off  SenseRad=off  SenseAzim=off  SenseDist=off  SenseInc=off  SenseXDot=off  SenseYDot=off  SenseZDot=off  SenseXYZDot=off  SenseRadDot=off  SenseAzimDot=off  SenseDistDot=off  SenseIncDot=off  SenseXDDot=off  SenseYDDot=off  SenseZDDot=off  SenseXYZDDot=off  SenseRadDDot=off  SenseAzimDDot=off  SenseDistDDot=off  SenseIncDDot=off
  ZScope : Scope
  force : Scope  NumInputPorts=2
  PlanB : PMIOPort  Side=Left
  SphF : PMIOPort  Port=2  Side=Right
  state : Outport  VectorParamsAs1DForOutWhenUnconnected=off
  wires:
  Sphere to Plane Force1/1 -> Bus Selector/1
  Bus Selector/1 -> force/1  "<Normal Force>"
  PSConv4/1 -> Compare To Constant/1, ZScope/1
  Compare To Constant/1 -> state/1, State Scope/1
  Bus Selector/3 -> force/2  "<Friction Force>"
  Bus Selector/2 -> Terminator/1  "<Frame Sep>"
  connections:
  Sphere to Plane Force1/LConn1 -- Transform Sensor/RConn1 -- SphF/RConn1
  Sphere to Plane Force1/RConn1 -- Transform Sensor/LConn1 -- PlanB/RConn1
  PSConv4/LConn1 -- Transform Sensor/RConn2

== system cambridge/quadruped robot plant/Contact_rr ==
  note: state 4 166.31ms
  note: 这是一个蛋疼的处理，因为地面现在厚度是0.4，为了和碰撞的block要求匹配，所以碰撞是相对于这个地面的中心来算的。而检测高度的时候就要把这个厚度减掉
      | 但是Transform sensor要检测的是球和地面的高度差
  Bus Selector : BusSelector  OutputSignals=Normal Force,Frame Sep,Friction Force
  Compare To Constant : simulink/Logic and Bit Operations/Compare To Constant  relop=<=  const=planner.touch_down_height  OutDataTypeStr=uint8
  PSConv4 : nesl_utility/PS-Simulink Converter  PhysicalDomain=network_engine_domain  SubClassName=ps_output  LeftPortType=input  RightPortType=output  PseudoPeriodic=off  Frequencies=[]  VectorFormat=1-D array  Unit=1  AffineConversion=off
  Sphere to Plane Force1 : Contact_Forces_Lib/3D/Sphere to Plane Force  sphere_rad=body.foot_radius  plane_lenx=12  plane_leny=12  plane_depth=0  force_law=Linear  k_contact=ground.stiff  b_contact=ground.damp  pen_full_damp_F=1e-4  pen_exponent=1  custom_param_1=1  custom_param_2=1  friction_law=Stick-Slip Continuous  mu_kinetic=0.7  mu_static=0.7  v_thr=0.001
  State Scope : Scope
  Terminator : Terminator
  Transform Sensor : sm_lib/Frames and Transforms/Transform Sensor  MeasurementFrame=World  RotationSequence=XYX  SenseAngle=off  SenseAxis=off  SenseQ=off  SenseR=off  SenseRotationSequence=off  SenseOmegaX=off  SenseOmegaY=off  SenseOmegaZ=off  SenseOmega=off  SenseQDot=off  SenseRDot=off  SenseRotationSequenceDot=off  SenseAlphaX=off  SenseAlphaY=off  SenseAlphaZ=off  SenseAlpha=off  SenseQDDot=off  SenseRDDot=off  SenseX=off  SenseY=off  SenseZ=on  SenseXYZ=off  SenseRad=off  SenseAzim=off  SenseDist=off  SenseInc=off  SenseXDot=off  SenseYDot=off  SenseZDot=off  SenseXYZDot=off  SenseRadDot=off  SenseAzimDot=off  SenseDistDot=off  SenseIncDot=off  SenseXDDot=off  SenseYDDot=off  SenseZDDot=off  SenseXYZDDot=off  SenseRadDDot=off  SenseAzimDDot=off  SenseDistDDot=off  SenseIncDDot=off
  ZScope : Scope
  force : Scope  NumInputPorts=2
  PlanB : PMIOPort  Side=Left
  SphF : PMIOPort  Port=2  Side=Right
  state : Outport  VectorParamsAs1DForOutWhenUnconnected=off
  wires:
  Sphere to Plane Force1/1 -> Bus Selector/1
  Bus Selector/1 -> force/1  "<Normal Force>"
  PSConv4/1 -> Compare To Constant/1, ZScope/1
  Compare To Constant/1 -> state/1, State Scope/1
  Bus Selector/3 -> force/2  "<Friction Force>"
  Bus Selector/2 -> Terminator/1  "<Frame Sep>"
  connections:
  Sphere to Plane Force1/LConn1 -- Transform Sensor/RConn1 -- SphF/RConn1
  Sphere to Plane Force1/RConn1 -- Transform Sensor/LConn1 -- PlanB/RConn1
  PSConv4/LConn1 -- Transform Sensor/RConn2

== system cambridge/quadruped robot plant/ground ==
  Mechanism Configuration : sm_lib/Utilities/Mechanism Configuration  UniformGravity=Constant  GravityVector=[0 0 -9.80665]  GravityVectorUnits=m/s^2  LinearizationDelta=0.001  JointModeTransitionNonlinearIterations=2
  Rigid Transform : sm_lib/Frames and Transforms/Rigid Transform  TranslationMethod=StandardAxis  TranslationStandardOffset=ground.height/2  TranslationStandardOffsetUnits=m  TranslationStandardAxis=+Z  TranslationCartesianOffset=[0 0 0]  TranslationCartesianOffsetUnits=m  TranslationROffset=0  TranslationROffsetUnits=m  TranslationZOffset=0  TranslationZOffsetUnits=m  TranslationThetaOffset=0  TranslationThetaOffsetUnits=deg  RotationMethod=None  RotationAngleUnits=deg  RotationStandardAxis=+Z  RotationAngle=0.0  RotationArbitraryAxis=[0 0 1]  FollAlignAxisA=+X  BaseAlignAxisA=+Y  FollAlignAxisB=+Y  BaseAlignAxisB=+Z  RotationSequenceAxes=FollowerAxes  RotationSequence=XYX  RotationSequenceAngles=[0 0 0]  RotationSequenceAnglesUnits=deg  RotationMatrix=[1 0 0; 0 1 0; 0 0 1]  Quaternion=[1 0 0 0]
  Solver Configuration : nesl_utility/Solver Configuration  PhysicalDomain=network_engine_domain  SubClassName=solver  LeftPortType=input  RightPortType=generic  Tones=[]  Harmonics=[]  SimulateNoise=off  Profile=off  UseLocalSampling=off  EnableSwitchedLinearOptims=on  FrequencyDomain=off  UseCCode=off  RelTol=0.001  AbsTol=1e-06  MinStep=1e-09  ToWorkspace=off  RevertToSquareIcSolve=off  NumHomotopyIterations=100  PhasorMode=off  PhasorModeNumHarmonics=1  ConsistencySolver=NEWTON_FTOL  IndexReductionMethod=DerivativeReplacement  DoDC=off  ResidualTolerance=1e-09  ConsistencyTolSource=GLOBAL  ConsistencyAbsTol=0.001  ConsistencyRelTol=0.001  ConsistencyTolFactor=0.001  UseLocalSolver=off  LocalSolverChoice=NE_BACKWARD_EULER_ADVANCER  ResolveIndetEquations=on  FunctionEvalNumThread=1  LocalSolverSampleTime=0.001  DoFixedCost=off  MaxNonlinIter=3  MaxModeIter=2  ComputeImpulses=off  ImpulseIterations=2  LinearAlgebra=Sparse  LinearAlgebraNumThread=0  EquationFormulation=NE_TIME_EF  DelaysMemoryBudget=1024  AutomaticFiltering=on  FilteringTimeConstant=0.001  PartitionStorageMethod=AS_NEEDED  PartitionMemoryBudget=1024  PartitionMethod=FAST  MultibodyUseLocalSolver=off  MultibodyLocalSolverChoice=ODE1  MultibodyLocalSolverSampleTime=0.001
  World Frame : sm_lib/Frames and Transforms/World Frame
  ground : sm_lib/Body Elements/Brick Solid  GraphicAmbientColor=[0.15 0.15 0.15 1.0]  BasedOnType=Density  BrickDimensions=[12 12 ground.height]  BrickDimensionsUnits=m  CenterOfMass=[0 0 0]  CenterOfMassUnits=m  GraphicDiffuseColor=[0.6 1.0 0.8]  Density=1000  DensityUnits=kg/(m^3)  DoExposeReferenceFrame=on  GraphicEmissiveColor=[0.0 0.0 0.0 1.0]  ExportEntireGeometry=off  SerializedFrames=<Frames/>  MarkerShape=Sphere  MarkerSize=10  GraphicType=FromGeometry  InertiaType=CalculateFromGeometry  Mass=1  MassUnits=kg  MomentsOfInertia=[1 1 1]  MomentsOfInertiaUnits=kg*m^2  GraphicOpacity=1.0  ProductsOfInertia=[0 0 0]  ProductsOfInertiaUnits=kg*m^2  GraphicShininess=75  GraphicSpecularColor=[0.5 0.5 0.5 1.0]  GraphicVisPropType=SimpleVisualProperties
  port1 : PMIOPort  Side=Right
  connections:
  Solver Configuration/RConn1 -- ground/RConn1 -- Mechanism Configuration/RConn1 -- Rigid Transform/LConn1 -- World Frame/RConn1
  port1/RConn1 -- Rigid Transform/RConn1
